simulink model "ex1"  (Simulink 5.0)
settings: Solver=ode45  StartTime=0.0  StopTime=10.0  RelTol=1e-3
settings Model: LastModifiedBy=alexandru

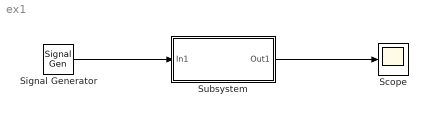
== system ex1 ==
  Scope : Scope
  Signal Generator : SignalGenerator
  Subsystem : Subsystem  mask{Kp=0.1, Kd=1, Ki=1}
      mask prompts: Kp "constelem prop"; Kd "const elem derivativ"; Ki "const elem integrator"
  wires:
  Signal Generator/1 -> Subsystem/1(In1)
  Subsystem/1(Out1) -> Scope/1

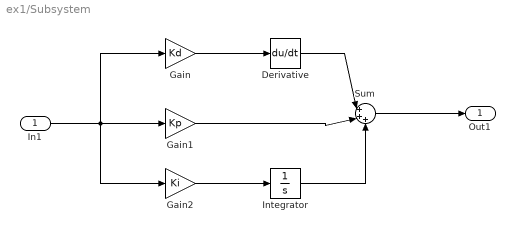
== system ex1/Subsystem ==
  In1 : Inport
  Derivative : Derivative
  Gain : Gain  Gain=Kd  SaturateOnIntegerOverflow=on
  Gain1 : Gain  Gain=Kp  SaturateOnIntegerOverflow=on
  Gain2 : Gain  Gain=Ki  SaturateOnIntegerOverflow=on
  Integrator : Integrator
  Sum : Sum  Inputs=|+++  SaturateOnIntegerOverflow=on
  Out1 : Outport
  wires:
  Derivative/1 -> Sum/1
  Integrator/1 -> Sum/3
  Gain1/1 -> Sum/2
  Sum/1 -> Out1/1
  Gain2/1 -> Integrator/1
  Gain/1 -> Derivative/1
  In1/1 -> Gain/1, Gain1/1, Gain2/1
